simulink model "rician_channel_sin"  (R2016b)
settings: Solver=FixedStepAuto  StartTime=0.0  StopTime=10^(-6)  FixedStep=2*10^(-11)  RelTol=1e-3  EnableMultiTasking=on
undefined symbols (not defined in the file): fdesignblkfcn, gcbh
libraries: simulink x2, commchan3 x2
settings Model: Creator=MOMENT OF PEACE  LastModifiedBy=MOMENT OF PEACE
settings DataIOCC: LimitDataPoints=on  SaveFormat=Array
settings OptimizationCC: LifeSpan=inf
settings DebuggingCC: SFUnexpectedBacktrackingDiag=warning  SFNoUnconditionalDefaultTransitionDiag=warning  SFExecutionAtInitializationDiag=none
settings HardwareCC: ProdBitPerPointer=32  ProdBitPerSizeT=32  ProdBitPerPtrDiffT=32  ProdLargestAtomicFloat=None  ProdIntDivRoundTo=Undefined  ProdEndianess=Unspecified  ProdWordSize=32  ProdHWDeviceType=32-bit Generic
settings ModelReferenceCC: PropagateSignalLabelsOutOfModel=off
settings GRTTargetCC: TargetLangStandard=C89/C90 (ANSI)  GeneratePreprocessorConditionals=Disable all
settings ConfigComp: CovMetricSettings=dw  CovHtmlReporting=on  CovSaveCumulativeToWorkspaceVar=on  CovSaveSingleToWorkspaceVar=on  CovExternalEMLEnable=off

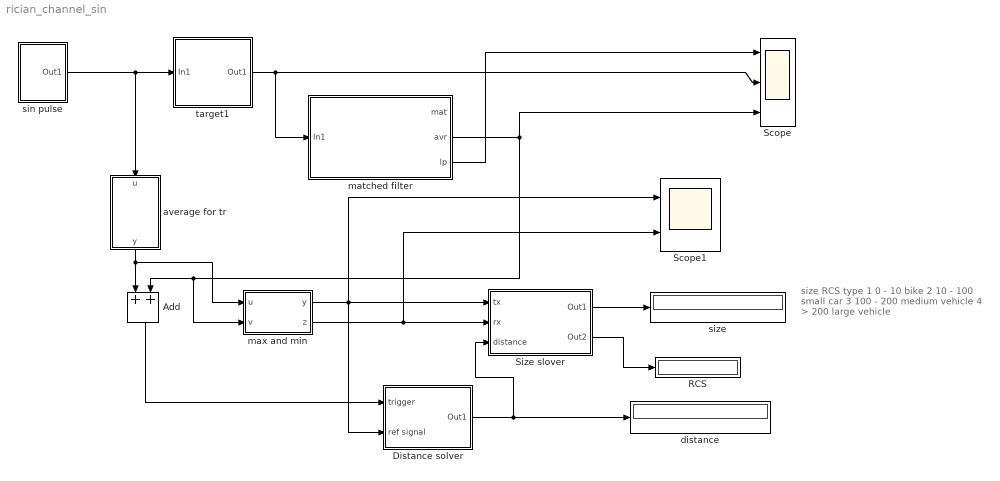
== system rician_channel_sin ==
  note: size RCS type
      | 1 0 - 10 bike
      | 2 10 - 100 small car
      | 3 100 - 200 medium vehicle
      | 4 > 200 large vehicle
  Add : Sum
  Distance solver : Subsystem
  RCS : Display
  Scope : Scope  NumInputPorts=3
  Scope1 : Scope  NumInputPorts=2
  Size slover : Subsystem
  average for tr : MATLAB Function  TreatAsAtomicUnit=on
  distance : Display
  matched filter : Subsystem
  max and min : MATLAB Function  TreatAsAtomicUnit=on
  sin pulse : Subsystem
  size : Display
  target1 : Subsystem  mask{d=25, v=10, s=240, snr=20, gain=10}
      mask prompts: d "Distance (m)"; v "Velocity (m/s)"; s "RCS (m^2)"; snr "SNR (dB)"; gain "Gain (dB)"
      mask init:
      | % d denotes the distance and v denotes velocity
      | c = 3e8;    % the speed of light
      | p = 1e-9;   % the width of impulse
      | r = 0.7;    % relectivity
      | rcs = s;
      | w = p * c;
      | 
      | G = 10^(gain/10);       % gain in decimal
      | delay = 2 * d / c;      % phase delay
      | loss = G^2 *  w^2 * rcs/((4 * pi)^3 * d^4);     % path loss
  wires:
  target1/1(Out1) -> Scope/2, matched filter/1(In1)
  matched filter/2(avr) -> Scope/3, max and min/2(v), Add/2
  sin pulse/1(Out1) -> target1/1(In1), average for tr/1(u)
  average for tr/1(y) -> max and min/1(u), Add/1
  Add/1 -> Distance solver/1(trigger)
  matched filter/3(lp) -> Scope/1
  max and min/1(y) -> Scope1/1, Size slover/1(tx), Distance solver/2(ref signal)
  Distance solver/1(Out1) -> Size slover/3(distance), distance/1
  max and min/2(z) -> Scope1/2, Size slover/2(rx)
  Size slover/1(Out1) -> size/1
  Size slover/2(Out2) -> RCS/1

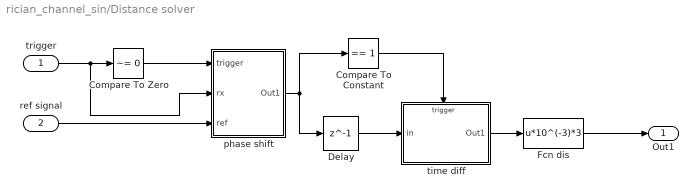
== system rician_channel_sin/Distance solver ==
  trigger : Inport
  ref signal : Inport  Port=2
  Compare To Constant : simulink/Logic and Bit Operations/Compare To Constant  relop===  const=1  OutDataTypeStr=boolean
  Compare To Zero : simulink/Logic and Bit Operations/Compare To Zero  relop=~=  OutDataTypeStr=uint8
  Delay : Delay  DelayLength=1  InitialCondition=0
  Fcn dis : Fcn  Expr=u*10^(-3)*3
  phase shift : Subsystem
  time diff : Subsystem  TreatAsAtomicUnit=on
  Out1 : Outport
  wires:
  ref signal/1 -> phase shift/3(ref)
  Fcn dis/1 -> Out1/1
  Compare To Constant/1 -> time diff/Trigger
  trigger/1 -> phase shift/2(rx), Compare To Zero/1
  time diff/1(Out1) -> Fcn dis/1
  Delay/1 -> time diff/1(in)
  phase shift/1(Out1) -> Compare To Constant/1, Delay/1
  Compare To Zero/1 -> phase shift/1(trigger)

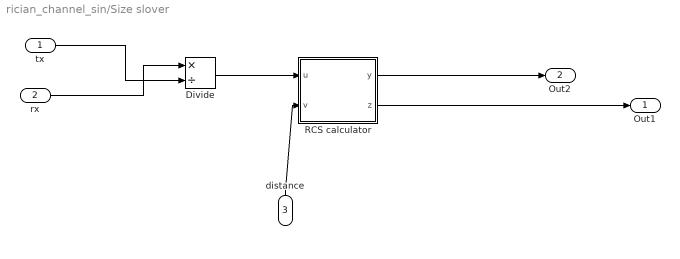
== system rician_channel_sin/Size slover ==
  tx : Inport
  rx : Inport  Port=2
  distance : Inport  Port=3
  Divide : Product  Inputs=*/
  RCS calculator : MATLAB Function  TreatAsAtomicUnit=on
  Out1 : Outport
  Out2 : Outport  Port=2
  wires:
  distance/1 -> RCS calculator/2(v)
  tx/1 -> Divide/2
  rx/1 -> Divide/1
  Divide/1 -> RCS calculator/1(u)
  RCS calculator/1(y) -> Out2/1
  RCS calculator/2(z) -> Out1/1

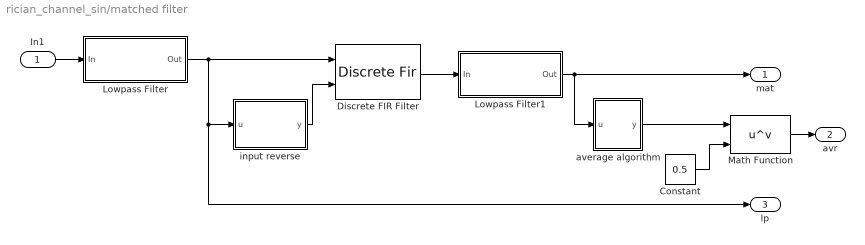
== system rician_channel_sin/matched filter ==
  In1 : Inport
  Constant : Constant  Value=0.5
  Discrete FIR Filter : DiscreteFir  CoefSource=Input port  Coefficients=[1 1 1 1 1 1]  InputProcessing=Columns as channels (frame based)
      settings: InputPortMap=u0,u1
  Lowpass Filter : Subsystem  DialogController=fdesignblkfcn  InitFcn=fdesignblkfcn(gcbh, {'InitFcn'});  mask(Lowpass Filter){}
      mask help: Design a lowpass filter
      settings: CopyFcn=fdesignblkfcn(gcbh, {'CopyFcn'});
      mask Help: helpview(mapfilelocation('dsp'), 'dsplowpassfilter');
      mask Display: disp('Lowpass')
  Lowpass Filter1 : Subsystem  DialogController=fdesignblkfcn  InitFcn=fdesignblkfcn(gcbh, {'InitFcn'});  mask(Lowpass Filter){}
      mask help: Design a lowpass filter
      settings: CopyFcn=fdesignblkfcn(gcbh, {'CopyFcn'});
      mask Help: helpview(mapfilelocation('dsp'), 'dsplowpassfilter');
      mask Display: disp('Lowpass')
  Math Function : Math  Operator=pow  SaturateOnIntegerOverflow=on
  average algorithm : MATLAB Function  TreatAsAtomicUnit=on
  input reverse : MATLAB Function  TreatAsAtomicUnit=on
  mat : Outport
  avr : Outport  Port=2
  lp : Outport  Port=3
  wires:
  In1/1 -> Lowpass Filter/1(In)
  input reverse/1(y) -> Discrete FIR Filter/2
  average algorithm/1(y) -> Math Function/1
  Discrete FIR Filter/1 -> Lowpass Filter1/1(In)
  Lowpass Filter/1(Out) -> Discrete FIR Filter/1, lp/1, input reverse/1(u)
  Lowpass Filter1/1(Out) -> mat/1, average algorithm/1(u)
  Math Function/1 -> avr/1
  Constant/1 -> Math Function/2

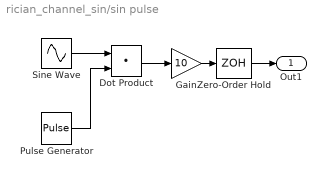
== system rician_channel_sin/sin pulse ==
  Dot Product : DotProduct  InputSameDT=on  OutDataTypeStr=Inherit: Inherit via internal rule
  Gain : Gain  Gain=10
  Pulse Generator : DiscretePulseGenerator  Amplitude=0.004  Period=15000  PulseWidth=500  SampleTime=2*10^(-11)
  Sine Wave : Sin  Frequency=1000000000*2*pi  SampleTime=0
  Zero-Order Hold : ZeroOrderHold  SampleTime=2*10^(-11)
  Out1 : Outport
  wires:
  Sine Wave/1 -> Dot Product/1
  Gain/1 -> Zero-Order Hold/1
  Dot Product/1 -> Gain/1
  Pulse Generator/1 -> Dot Product/2
  Zero-Order Hold/1 -> Out1/1

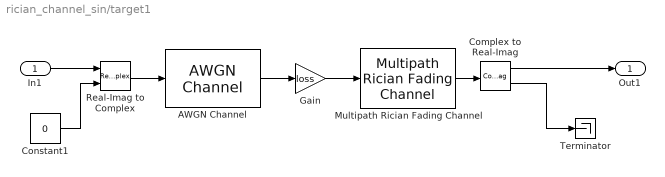
== system rician_channel_sin/target1 ==
  In1 : Inport
  AWGN Channel : commchan3/AWGN Channel  InputProcessing=Columns as channels (frame based)  seed=67  noiseMode="Signal to noise ratio  (SNR)"  EbNodB=10  EsNodB=10  SNRdB=snr  bitsPerSym=1  Ps=0.004/300  Tsym=1  variance=1
  Complex to Real-Imag : ComplexToRealImag
  Constant1 : Constant  Value=0
  Gain : Gain  Gain=loss
  Multipath Rician Fading Channel : commchan3/Multipath Rician Fading Channel  K=100  fdLOS=0  thetaLOS=0  maxDopplerShift=40  spectrumType=Jakes  sigmaGaussian=1/sqrt(2)  coeffRounded=[1 -1.72 0.785]  freqMinMaxRJakes=[0 1]  freqMinMaxAJakes=[0 1]  sigmaGaussian1=1/sqrt(2)  sigmaGaussian2=1/sqrt(2)  centerFreqGaussian1=0  centerFreqGaussian2=0  gainGaussian1=0.5  gainGaussian2=0.5  coeffBell=9  dopplerSpectrum=doppler.jakes  pathDelays=[delay delay+(5e-8) delay+(1e-7)]  avgPathGaindB=[0 -1 -1]  normalizePathGains=on  seed=73  enableProbe=0  openVisAtStart=off  outPathGains=off  outDelay=off
  Real-Imag to Complex : RealImagToComplex
  Terminator : Terminator
  Out1 : Outport
  wires:
  Complex to Real-Imag/1 -> Out1/1
  AWGN Channel/1 -> Gain/1
  Multipath Rician Fading Channel/1 -> Complex to Real-Imag/1
  Constant1/1 -> Real-Imag to Complex/2
  In1/1 -> Real-Imag to Complex/1
  Complex to Real-Imag/2 -> Terminator/1
  Real-Imag to Complex/1 -> AWGN Channel/1
  Gain/1 -> Multipath Rician Fading Channel/1

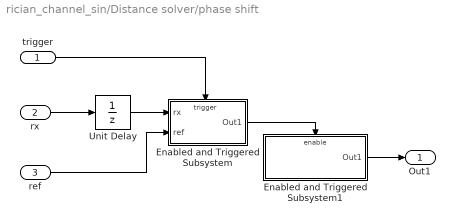
== system rician_channel_sin/Distance solver/phase shift ==
  trigger : Inport
  rx : Inport  Port=2
  ref : Inport  Port=3
  Enabled and Triggered Subsystem : Subsystem  TreatAsAtomicUnit=on
  Enabled and Triggered Subsystem1 : Subsystem  TreatAsAtomicUnit=on
  Unit Delay : UnitDelay  SampleTime=-1
  Out1 : Outport
  wires:
  Enabled and Triggered Subsystem/1(Out1) -> Enabled and Triggered Subsystem1/Enable
  trigger/1 -> Enabled and Triggered Subsystem/Trigger
  Enabled and Triggered Subsystem1/1(Out1) -> Out1/1
  rx/1 -> Unit Delay/1
  ref/1 -> Enabled and Triggered Subsystem/2(ref)
  Unit Delay/1 -> Enabled and Triggered Subsystem/1(rx)

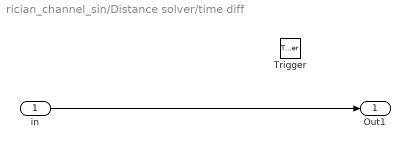
== system rician_channel_sin/Distance solver/time diff ==
  in : Inport
  Trigger : TriggerPort  VariantControl=Variant  ZeroCross=off
  Out1 : Outport
  wires:
  in/1 -> Out1/1

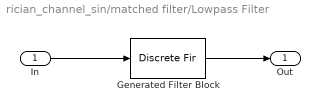
== system rician_channel_sin/matched filter/Lowpass Filter ==
  In : Inport
  Generated Filter Block : DiscreteFir  Tag=BlockMethodSubSystem  Coefficients=[-0.00882242952209379323 -0.00250396131135136295 0.0203488178406029327 0.00845153638179320724 -0.00156508516764006927 0.0105860024294243335 -0.00352454868452364151 0.00077576045905514146 0.00717622040828255932 -0.00940111963814425564 0.00797382618152611515 -0.000273978864866431318 -0.00850196312346529828 0.0141906978084733945 -0.0119506479715848612 0.00181855656901186435 0.0118184144727089858 -0.0210959922579116305 0.0193002857308069292 -0.00470681791085527865 -0.0167959060315205945 0.0337033448793372867 -0.0339636229705798098 0.0118324414990105195 0.0272315640460091407 -0.0660974718487657292 0.0800981455589089425 -0.0421164040979259552 -0.0871991530250003505 0.590547367711231064 0.590547367711231064 -0.0871991530250003505 -0.0421164040979259552 0.0800981455589089425 -0.0660974718487657292 0.0272315640460091407 0.0118324414990105195 -0.0339636229705798098 0.0337033448793372867 -0.0167959060315205945 -0.00470681791085527865 0.0193002857308069292 -0.0210959922579116305 0.0118184144727089858 0.00181855656901186435 -0.0119506479715848612 0.0141906978084733945 -0.00850196312346529828 -0.000273978864866431318 0.00797382618152611515 -0.00940111963814425564 0.00717622040828255932 0.00077576045905514146 -0.00352454868452364151 0.0105860024294243335 -0.00156508516764006927 0.00845153638179320724 0.0203488178406029327 -0.00250396131135136295 -0.00882242952209379323]  InputProcessing=Columns as channels (frame based)
  Out : Outport
  wires:
  In/1 -> Generated Filter Block/1
  Generated Filter Block/1 -> Out/1

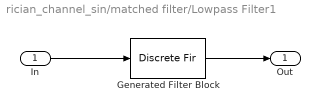
== system rician_channel_sin/matched filter/Lowpass Filter1 ==
  In : Inport
  Generated Filter Block : DiscreteFir  Tag=BlockMethodSubSystem  Coefficients=[-0.00882242952209379323 -0.00250396131135136295 0.0203488178406029327 0.00845153638179320724 -0.00156508516764006927 0.0105860024294243335 -0.00352454868452364151 0.00077576045905514146 0.00717622040828255932 -0.00940111963814425564 0.00797382618152611515 -0.000273978864866431318 -0.00850196312346529828 0.0141906978084733945 -0.0119506479715848612 0.00181855656901186435 0.0118184144727089858 -0.0210959922579116305 0.0193002857308069292 -0.00470681791085527865 -0.0167959060315205945 0.0337033448793372867 -0.0339636229705798098 0.0118324414990105195 0.0272315640460091407 -0.0660974718487657292 0.0800981455589089425 -0.0421164040979259552 -0.0871991530250003505 0.590547367711231064 0.590547367711231064 -0.0871991530250003505 -0.0421164040979259552 0.0800981455589089425 -0.0660974718487657292 0.0272315640460091407 0.0118324414990105195 -0.0339636229705798098 0.0337033448793372867 -0.0167959060315205945 -0.00470681791085527865 0.0193002857308069292 -0.0210959922579116305 0.0118184144727089858 0.00181855656901186435 -0.0119506479715848612 0.0141906978084733945 -0.00850196312346529828 -0.000273978864866431318 0.00797382618152611515 -0.00940111963814425564 0.00717622040828255932 0.00077576045905514146 -0.00352454868452364151 0.0105860024294243335 -0.00156508516764006927 0.00845153638179320724 0.0203488178406029327 -0.00250396131135136295 -0.00882242952209379323]  InputProcessing=Columns as channels (frame based)
  Out : Outport
  wires:
  Generated Filter Block/1 -> Out/1
  In/1 -> Generated Filter Block/1

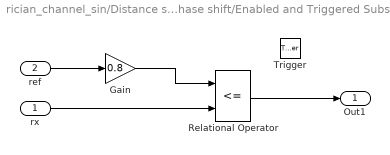
== system rician_channel_sin/Distance solver/phase shift/Enabled and Triggered Subsystem ==
  rx : Inport
  ref : Inport  Port=2
  Trigger : TriggerPort  TriggerType=falling  VariantControl=Variant
  Gain : Gain  Gain=0.8
  Relational Operator : RelationalOperator  Operator=<=  OutDataTypeStr=boolean  RndMeth=Nearest
  Out1 : Outport
  wires:
  ref/1 -> Gain/1
  Gain/1 -> Relational Operator/1
  rx/1 -> Relational Operator/2
  Relational Operator/1 -> Out1/1

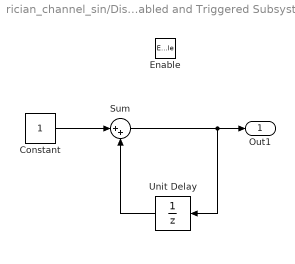
== system rician_channel_sin/Distance solver/phase shift/Enabled and Triggered Subsystem1 ==
  Enable : EnablePort  StatesWhenEnabling=reset
  Constant : Constant
  Sum : Sum  Inputs=|++
  Unit Delay : UnitDelay  SampleTime=-1
  Out1 : Outport
  wires:
  Constant/1 -> Sum/1
  Sum/1 -> Unit Delay/1, Out1/1
  Unit Delay/1 -> Sum/2

== matlab function rician_channel_sin/matched filter/average algorithm ==
  data: u input; y output
function y = fcn(u)
%#codegen
persistent summ;
persistent maxm;
n = 200;

if isempty(maxm)
    maxm = -1;
end

if isempty(summ)
    summ = zeros(1,n);
end

if u > max(summ)
    maxm = u;
end

if (u < 0.7*maxm)
    y = 0;
else
    summ = circshift(summ,[0,1]);
    summ(1) = u;
    y = sum(summ) / n;
end

== matlab function rician_channel_sin/matched filter/input reverse ==
  data: u input; y output
function y = fcn(u)
%#codegen

y = u(end:-1:1);

== matlab function rician_channel_sin/average for tr ==
  data: u input; y output
function y = fcn(u)
%#codegen
persistent sum;
persistent n;
persistent maxm;

if isempty(maxm)
    maxm = -1;
end

if isempty(sum)
    sum = 0;
end

if isempty(n)
    n = 0;
end

if u > maxm
    maxm = u;
end

if (u < 0.7*maxm)
    y = 0;
else
    sum = sum + u;
    n = n + 1;
    y = sum / n;
end

== matlab function rician_channel_sin/max and min ==
  data: u input; y output; v input; z output
function [y,z] = fcn(u,v)
%#codegen
persistent maxm;
persistent minm;

if isempty(maxm)
    maxm = -1;
end

if isempty(minm)
    minm = -1;
end

if u > 0
    maxm = u;
end

if v > 0
    minm = v;
end

y = maxm;
z = minm;

== matlab function rician_channel_sin/Size slover/RCS calculator ==
  data: u input; y output; v input; z output
function [y,z] = fcn(u,v)
%#codegen
G = 10;
w = 0.3;
y = 1.69 * u * ((4 * pi)^3 * v^4)/(G^2 *  w^2);
if y < 10
    z = 1;%'bike';
elseif y < 100
    z = 2;%'small car';
elseif y < 200
    z = 3;%'SUV or small truck';
else
    z = 4;%'truck';
end
